simulink model "Proyecto01"  (R2017a)
settings: Solver=VariableStepAuto  StartTime=0.0  StopTime=300  RelTol=1e-3
undefined symbols (not defined in the file or in its folder): dfilt
libraries: dsparch4 x7, dspvision x2, dspsrcs4 x1, dspobslib x1
settings Model: Creator=ITAM\mmejiam  LastModifiedBy=LFERNANDAY

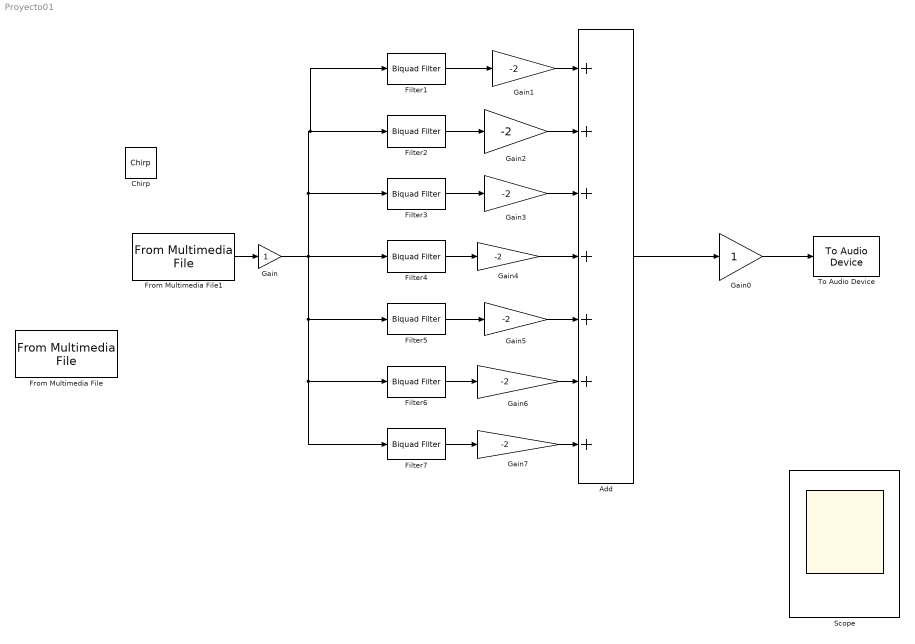
== system Proyecto01 ==
  Add : Sum  Inputs=+++++++
  Chirp : dspsrcs4/Chirp  sweep=Logarithmic  mode=Unidirectional  f0=50  f1=16000  t1=1  Tsweep=1  phase=0  Ts=1/44100  spf=1  datatype=Single  OutputFrames=on
      settings: SourceProductName=DSP System Toolbox
  Filter1 : dsparch4/Biquad Filter  Tag=BlockMethodSubSystem  IIRFiltStruct=Direct form II  CoeffSource=Specify via dialog  BiQuadCoeffs=[1 2 1 1 -1.9885375869222708 0.98866676530711495;1 1 0 1 -0.98866639929305644 0]  a0Flag=Warning  IC=0  ICnum=0  ICden=0  InputProcessing=Columns as channels (frame based)  denAccumFracLength=30  denProdOutputFracLength=30  secondMemoryFracLength=15  roundingMode=Floor  overflowMode=off  ScaleValues=[3.2294596211033898e-05;0.0056668003534717784;1]  optimizeScaleValues=on  ScaleValueMode=Specify via input port (g)  scaleValueFracLength=14  FilterSource=Specify via dialog  FilterObject=dfilt.df2tsos([1 0.3 0.4],[1 0.1 0.2])
      settings: SourceProductName=DSP System Toolbox
  Filter2 : dsparch4/Biquad Filter  Tag=BlockMethodSubSystem  IIRFiltStruct=Direct form II  CoeffSource=Specify via dialog  BiQuadCoeffs=[1 0 -1 1 -1.984628508680776 0.98559222359592769;1 0 -1 1 -1.9938491816920214 0.9940147559084499;1 0 -1 1 -1.9792936532423133 0.9796910981914434]  a0Flag=Warning  IC=0  ICnum=0  ICden=0  InputProcessing=Columns as channels (frame based)  denAccumFracLength=30  denProdOutputFracLength=30  secondMemoryFracLength=15  roundingMode=Floor  overflowMode=off  ScaleValues=[0.010205871776313696;0.010205871776313696;0.010154450904278245;1]  optimizeScaleValues=on  ScaleValueMode=Specify via input port (g)  scaleValueFracLength=14  FilterSource=Specify via dialog  FilterObject=dfilt.df2tsos([1 0.3 0.4],[1 0.1 0.2])
      settings: SourceProductName=DSP System Toolbox
  Filter3 : dsparch4/Biquad Filter  Tag=BlockMethodSubSystem  IIRFiltStruct=Direct form II  CoeffSource=Specify via dialog  BiQuadCoeffs=[1 0 -1 1 -1.961922591681837 0.9684871642054973;1 0 -1 1 -1.9830018692291436 0.98456249731394352;1 0 -1 1 -1.9503462238792653 0.95351043820588]  a0Flag=Warning  IC=0  ICnum=0  ICden=0  InputProcessing=Columns as channels (frame based)  denAccumFracLength=30  denProdOutputFracLength=30  secondMemoryFracLength=15  roundingMode=Floor  overflowMode=off  ScaleValues=[0.023513241192071255;0.023513241192071255;0.023244780897059975;1]  optimizeScaleValues=on  ScaleValueMode=Specify via input port (g)  scaleValueFracLength=14  FilterSource=Specify via dialog  FilterObject=dfilt.df2tsos([1 0.3 0.4],[1 0.1 0.2])
      settings: SourceProductName=DSP System Toolbox
  Filter4 : dsparch4/Biquad Filter  Tag=BlockMethodSubSystem  IIRFiltStruct=Direct form II  CoeffSource=Specify via dialog  BiQuadCoeffs=[1 0 -1 1 -1.8494047291540761 0.89747972026414202;1 0 -1 1 -1.949588343291264 0.95750831590889218;1 0 -1 1 -1.8397266763195375 0.85858760326504902]  a0Flag=Warning  IC=0  ICnum=0  ICden=0  InputProcessing=Columns as channels (frame based)  denAccumFracLength=30  denProdOutputFracLength=30  secondMemoryFracLength=15  roundingMode=Floor  overflowMode=off  ScaleValues=[0.0731502644918781;0.0731502644918781;0.070706198367475465;1]  optimizeScaleValues=on  ScaleValueMode=Specify via input port (g)  scaleValueFracLength=14  FilterSource=Specify via dialog  FilterObject=dfilt.df2tsos([1 0.3 0.4],[1 0.1 0.2])
      settings: SourceProductName=DSP System Toolbox
  Filter5 : dsparch4/Biquad Filter  Tag=BlockMethodSubSystem  IIRFiltStruct=Direct form II  CoeffSource=Specify via dialog  BiQuadCoeffs=[1 0 -1 1 -1.5923541991504684 0.81632637473844172;1 0 -1 1 -1.8555819452158495 0.90728230022726775;1 0 -1 1 -1.634163695229059 0.73540691073313624]  a0Flag=Warning  IC=0  ICnum=0  ICden=0  InputProcessing=Columns as channels (frame based)  denAccumFracLength=30  denProdOutputFracLength=30  secondMemoryFracLength=15  roundingMode=Floor  overflowMode=off  ScaleValues=[0.1406132895072727;0.1406132895072727;0.13229654463343191;1]  optimizeScaleValues=on  ScaleValueMode=Specify via input port (g)  scaleValueFracLength=14  FilterSource=Specify via dialog  FilterObject=dfilt.df2tsos([1 0.3 0.4],[1 0.1 0.2])
      settings: SourceProductName=DSP System Toolbox
  Filter6 : dsparch4/Biquad Filter  Tag=BlockMethodSubSystem  IIRFiltStruct=Direct form II  CoeffSource=Specify via dialog  BiQuadCoeffs=[1 0 -1 1 -1.4957640580632705 0.75721498805346343;1 0 -1 1 -0.36524604746555162 0.59205366017181826;1 0 -1 1 -0.86626730728216894 0.36766753949124337]  a0Flag=Warning  IC=0  ICnum=0  ICden=0  InputProcessing=Columns as channels (frame based)  denAccumFracLength=30  denProdOutputFracLength=30  secondMemoryFracLength=15  roundingMode=Floor  overflowMode=off  ScaleValues=[0.35712008549469304;0.35712008549469304;0.31616623025437834;1]  optimizeScaleValues=on  ScaleValueMode=Specify via input port (g)  scaleValueFracLength=14  FilterSource=Specify via dialog  FilterObject=dfilt.df2tsos([1 0.3 0.4],[1 0.1 0.2])
      settings: SourceProductName=DSP System Toolbox
  Filter7 : dsparch4/Biquad Filter  Tag=BlockMethodSubSystem  IIRFiltStruct=Direct form II  CoeffSource=Specify via dialog  BiQuadCoeffs=[1 -2 1 1 0.18521823044240202 0.33762847553681591;1 -1 0 1 0.069568889518433236 0]  a0Flag=Warning  IC=0  ICnum=0  ICden=0  InputProcessing=Columns as channels (frame based)  denAccumFracLength=30  denProdOutputFracLength=30  secondMemoryFracLength=15  roundingMode=Floor  overflowMode=off  ScaleValues=[0.28810256127360345;0.46521555524078334;1]  optimizeScaleValues=on  ScaleValueMode=Specify via input port (g)  scaleValueFracLength=14  FilterSource=Specify via dialog  FilterObject=dfilt.df2tsos([1 0.3 0.4],[1 0.1 0.2])
      settings: SourceProductName=DSP System Toolbox
  From Multimedia File : dspvision/From Multimedia File  inputFilename=C:\Users\LFERNANDAY\Downloads\Proyecto01\My_Hero_Academia_-_You_Say_Run_(mp3.pm).mp3  loop=on  numPlays=1  outputStreams=Audio only  videoDataType=single  audioDataType=double  inheritSampleTime=on  userDefinedSampleTime=1/30  noAudioOutput=off  isIntensityVideo=off  fourcc=RGB  colorVideoFormat=Separate color signals  outputEOF=off  dataOrg=Column-major  audioFrameSize=44100  computeAudioFrameSize=off  outSamplingMode=Sample based
      settings: SourceProductBaseCode=VP
  From Multimedia File1 : dspvision/From Multimedia File  inputFilename=C:\Users\LFERNANDAY\Downloads\Proyecto01\Bohemian_Rhapsody_Audio_Only[ListenVid.com].mp3  loop=on  numPlays=1  outputStreams=Audio only  videoDataType=single  audioDataType=double  inheritSampleTime=on  userDefinedSampleTime=1/30  noAudioOutput=off  isIntensityVideo=off  fourcc=RGB  colorVideoFormat=Separate color signals  outputEOF=off  dataOrg=Column-major  audioFrameSize=44100  computeAudioFrameSize=off  outSamplingMode=Sample based
      settings: SourceProductBaseCode=VP
  Gain : Gain
  Gain0 : Gain
  Gain{1..7} (7 alike) : Gain  Gain=-2
  Scope : Scope  NumInputPorts=2
  To Audio Device : dspobslib/To Audio Device  deviceName=Altavoz/Auricular (Realtek High Definition Audio)  inheritSampleRate=on  sampleRate=44100  deviceDatatype=Determine from input data type  autoBufferSize=on  bufferSize=4096  queueDuration=1.0  defaultOutputChannelMapping=on  outputChannelMapping=1:2  outputNumUnderrunSamples=off
      settings: SourceProductName=DSP System Toolbox  SourceProductBaseCode=DS
  wires:
  Gain1/1 -> Add/1
  Gain3/1 -> Add/3
  Gain4/1 -> Add/4
  Gain5/1 -> Add/5
  Gain6/1 -> Add/6
  Gain7/1 -> Add/7
  Gain2/1 -> Add/2
  Filter1/1 -> Gain1/1
  Filter2/1 -> Gain2/1
  Filter3/1 -> Gain3/1
  Filter7/1 -> Gain7/1
  Filter6/1 -> Gain6/1
  Filter5/1 -> Gain5/1
  Filter4/1 -> Gain4/1
  Gain0/1 -> To Audio Device/1
  Add/1 -> Gain0/1
  Gain/1 -> Filter1/1, Filter2/1, Filter3/1, Filter4/1, Filter5/1, Filter6/1, Filter7/1
  From Multimedia File1/1 -> Gain/1
